simulink model "controlador_slotine_li"  (R2021a)
settings: Solver=ode15s  StartTime=0.0  StopTime=2*pi  RelTol=1e-3
model workspace (MAT data in the model file):
  K_d = 5
  lambda = 10
  wn = 3.14159265359
libraries: roblocks x4
settings Model: Creator=Lucas  LastModifiedBy=Lucas

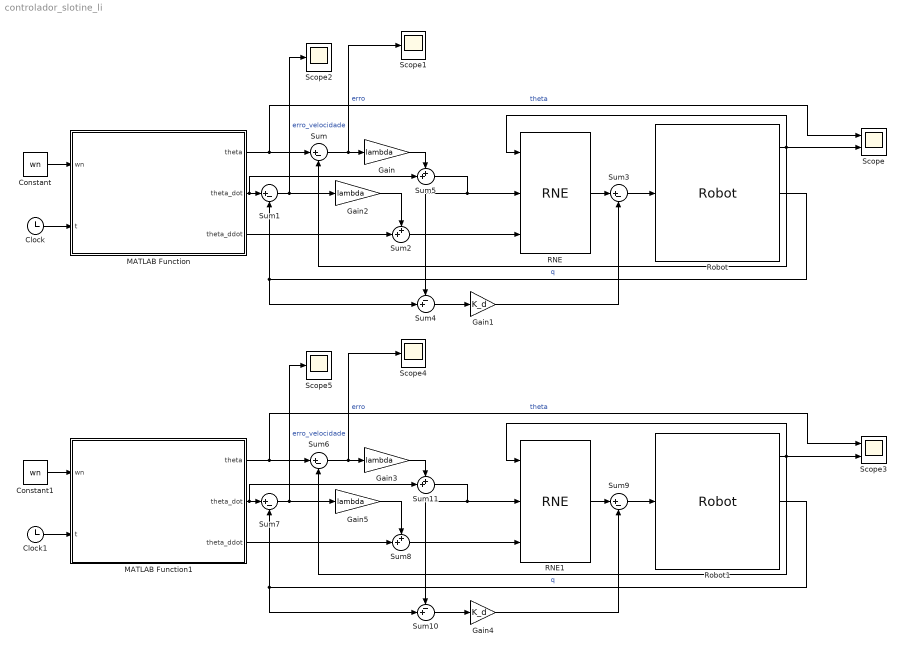
== system controlador_slotine_li ==
  Clock : Clock
  Clock1 : Clock
  Constant : Constant  Value=wn
  Constant1 : Constant  Value=wn
  Gain{,2..3,5} (4 alike) : Gain  Gain=lambda
  Gain1 : Gain  Gain=K_d
  Gain4 : Gain  Gain=K_d
  MATLAB Function : MATLAB Function  TreatAsAtomicUnit=on
  MATLAB Function1 : MATLAB Function  TreatAsAtomicUnit=on
  RNE : roblocks/Arm/RNE  robot=kinova  grav=[0 0 9.81]
  RNE1 : roblocks/Arm/RNE  robot=kinova  grav=[0 0 9.81]
  Robot : roblocks/Arm/Robot  robot=kinova  q0=deg2rad([0, 15, 180, -130, 0, 55, 90])
  Robot1 : roblocks/Arm/Robot  robot=kinova_alterado  q0=deg2rad([0, 15, 180, -130, 0, 55, 90])
  Scope : Scope  NumInputPorts=2
  Scope{1..2,4..5} (4 alike) : Scope
  Scope3 : Scope  NumInputPorts=2
  Sum{,1,3,6..7,9} (6 alike) : Sum  Inputs=|+-
  Sum10 : Sum  Inputs=-+|
  Sum{2,5,8,11} (4 alike) : Sum  Inputs=++|
  Sum4 : Sum  Inputs=-+|
  wires:
  Constant/1 -> MATLAB Function/1(wn)
  Clock/1 -> MATLAB Function/2(t)
  MATLAB Function/2(theta_dot) -> Sum5/2, Sum1/1
  MATLAB Function/1(theta) -> Scope/1, Sum/1  "theta"
  Robot/1 -> RNE/1, Scope/2, Sum/2  "q"
  Robot/2 -> Sum4/2, Sum1/2
  Sum/1 -> Gain/1, Scope1/1  "erro"
  Sum1/1 -> Gain2/1, Scope2/1  "erro_velocidade"
  Gain/1 -> Sum5/1
  RNE/1 -> Sum3/1
  Sum3/1 -> Robot/1
  Sum4/1 -> Gain1/1
  Gain1/1 -> Sum3/2
  MATLAB Function/3(theta_ddot) -> Sum2/2
  Sum2/1 -> RNE/3
  Gain2/1 -> Sum2/1
  Sum5/1 -> RNE/2, Sum4/1
  Sum11/1 -> RNE1/2, Sum10/1
  Robot1/1 -> RNE1/1, Scope3/2, Sum6/2  "q"
  Sum7/1 -> Gain5/1, Scope5/1  "erro_velocidade"
  Gain4/1 -> Sum9/2
  Sum8/1 -> RNE1/3
  MATLAB Function1/2(theta_dot) -> Sum11/2, Sum7/1
  Sum10/1 -> Gain4/1
  Sum9/1 -> Robot1/1
  MATLAB Function1/3(theta_ddot) -> Sum8/2
  Constant1/1 -> MATLAB Function1/1(wn)
  RNE1/1 -> Sum9/1
  Gain3/1 -> Sum11/1
  Sum6/1 -> Gain3/1, Scope4/1  "erro"
  Gain5/1 -> Sum8/1
  Clock1/1 -> MATLAB Function1/2(t)
  MATLAB Function1/1(theta) -> Scope3/1, Sum6/1  "theta"
  Robot1/2 -> Sum10/2, Sum7/2

== matlab function controlador_slotine_li/MATLAB Function1 ==
  data: wn input; theta output; t input; theta_dot output; theta_ddot output
function [theta, theta_dot, theta_ddot] = trajetoria_desejada(wn, t)
    % Função para calcular a trajetória desejada e suas derivadas
    
    % Trajetórias desejadas (em radianos)
    theta = [
        0.5236 * cos(wn * t);                              % θ1d
        0.2618 + 0.2618 * cos(wn * t);                     % θ2d (1)
        pi * ones(size(t));                                % θ2d (2)
        -2.2689 + 0.2618 * cos(1.2 * wn * t);              % θ2d (3)
        zeros(size(t));                                    % θ2d (4)
        0.9599 + 0.2618 * cos(1.3 * wn * t);               % θ2d (5)
        pi/2 * ones(size(t));                              % θ2d (6)
    ];
    
    % Primeira derivada das trajetórias
    theta_dot = [
        -0.5236 * wn * sin(wn * t);                        % θ1d_dot
        -0.2618 * wn * sin(wn * t);                        % θ2d_dot (1)
        zeros(size(t));                                    % θ2d_dot (2)
        -0.2618 * 1.2 * wn * sin(1.2 * wn * t);            % θ2d_dot (3)
        zeros(size(t));                                    % θ2d_dot (4)
        -0.2618 * 1.3 * wn * sin(1.3 * wn * t);            % θ2d_dot (5)
        zeros(size(t));                                    % θ2d_dot (6)
    ];
    
    % Segunda derivada das trajetórias
    theta_ddot = [
        -0.5236 * wn^2 * cos(wn * t);                      % θ1d_ddot
        -0.2618 * wn^2 * cos(wn * t);                      % θ2d_ddot (1)
        zeros(size(t));                                    % θ2d_ddot (2)
        -0.2618 * (1.2 * wn)^2 * cos(1.2 * wn * t);        % θ2d_ddot (3)
        zeros(size(t));                                    % θ2d_ddot (4)
        -0.2618 * (1.3 * wn)^2 * cos(1.3 * wn * t);        % θ2d_ddot (5)
        zeros(size(t));                                    % θ2d_ddot (6)
    ];
end

== matlab function controlador_slotine_li/MATLAB Function ==
  data: wn input; theta output; t input; theta_dot output; theta_ddot output
function [theta, theta_dot, theta_ddot] = trajetoria_desejada(wn, t)
    % Função para calcular a trajetória desejada e suas derivadas
    
    % Trajetórias desejadas (em radianos)
    theta = [
        0.5236 * cos(wn * t);                              % θ1d
        0.2618 + 0.2618 * cos(wn * t);                     % θ2d (1)
        pi * ones(size(t));                                % θ2d (2)
        -2.2689 + 0.2618 * cos(1.2 * wn * t);              % θ2d (3)
        zeros(size(t));                                    % θ2d (4)
        0.9599 + 0.2618 * cos(1.3 * wn * t);               % θ2d (5)
        pi/2 * ones(size(t));                              % θ2d (6)
    ];
    
    % Primeira derivada das trajetórias
    theta_dot = [
        -0.5236 * wn * sin(wn * t);                        % θ1d_dot
        -0.2618 * wn * sin(wn * t);                        % θ2d_dot (1)
        zeros(size(t));                                    % θ2d_dot (2)
        -0.2618 * 1.2 * wn * sin(1.2 * wn * t);            % θ2d_dot (3)
        zeros(size(t));                                    % θ2d_dot (4)
        -0.2618 * 1.3 * wn * sin(1.3 * wn * t);            % θ2d_dot (5)
        zeros(size(t));                                    % θ2d_dot (6)
    ];
    
    % Segunda derivada das trajetórias
    theta_ddot = [
        -0.5236 * wn^2 * cos(wn * t);                      % θ1d_ddot
        -0.2618 * wn^2 * cos(wn * t);                      % θ2d_ddot (1)
        zeros(size(t));                                    % θ2d_ddot (2)
        -0.2618 * (1.2 * wn)^2 * cos(1.2 * wn * t);        % θ2d_ddot (3)
        zeros(size(t));                                    % θ2d_ddot (4)
        -0.2618 * (1.3 * wn)^2 * cos(1.3 * wn * t);        % θ2d_ddot (5)
        zeros(size(t));                                    % θ2d_ddot (6)
    ];
end
